simulink model "Clik_Jacobian_pseudoinverse"  (R2023b)
settings: Solver=VariableStepAuto  StartTime=0.0  StopTime=20  RelTol=1e-3
undefined symbols (not defined in the file): DiscIntNeverNeededParam, f_s
settings Model: Creator=Gianluca  LastModifiedBy=ANDREA
settings OptimizationCC: ReuseModelBlockBuffer=off
settings ModelReferenceCC: EnableRefExpFcnMdlSchedulingChecks=on

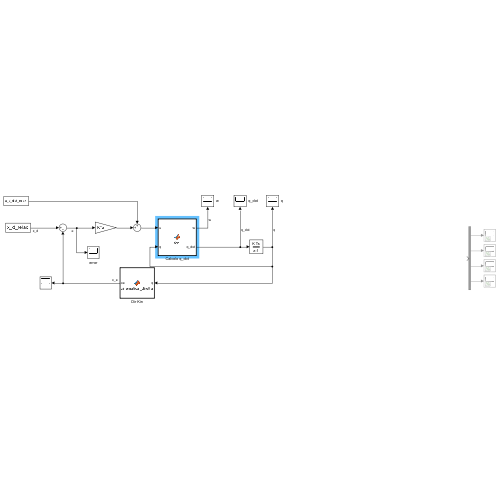
[thumbnail: Simulink's stored preview of the top-level diagram]
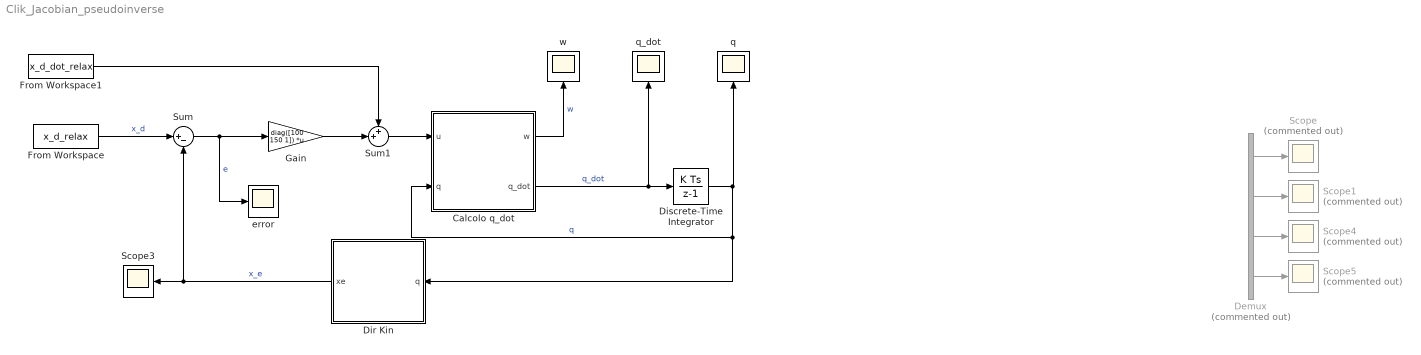
== system Clik_Jacobian_pseudoinverse ==
  "Calcolo q_dot " : MATLAB Function  TreatAsAtomicUnit=on
  Demux : Demux  Commented=on
  Dir Kin : MATLAB Function  TreatAsAtomicUnit=on
  Discrete-Time Integrator : DiscreteIntegrator  InitialCondition=[1.07216, -1.5708, 0.2, -0.49864 ]  SampleTime=1/f_s  ICPrevOutput=DiscIntNeverNeededParam  ICPrevScaledInput=DiscIntNeverNeededParam
  From Workspace : FromWorkspace  VariableName=x_d_relax  OutputAfterFinalValue=Holding final value
  From Workspace1 : FromWorkspace  VariableName=x_d_dot_relax
  Gain : Gain  Gain=diag([100 150 1])  Multiplication=Matrix(K*u)
  Scope{,1,4..5} (4 alike) : Scope  Commented=on
  Scope3 : Scope
  Sum : Sum  Inputs=|+-
  Sum1 : Sum  Inputs=++|
  error : Scope
  q : Scope
  q_dot : Scope
  w : Scope
  wires:
  Discrete-Time Integrator/1 -> q/1, Dir Kin/1(q), "Calcolo q_dot "/2(q)  "q"
  Gain/1 -> Sum1/2
  Sum1/1 -> "Calcolo q_dot "/1(u)
  "Calcolo q_dot "/2(q_dot) -> q_dot/1, Discrete-Time Integrator/1  "q_dot"
  Demux/1 -> Scope/1
  Demux/2 -> Scope1/1
  Demux/3 -> Scope4/1
  Sum/1 -> error/1, Gain/1  "e"
  "Calcolo q_dot "/1(w) -> w/1  "w"
  From Workspace/1 -> Sum/1  "x_d"
  Dir Kin/1(xe) -> Scope3/1, Sum/2  "x_e"
  Demux/4 -> Scope5/1
  From Workspace1/1 -> Sum1/1

== matlab function Clik_Jacobian_pseudoinverse/Calcolo q_dot  ==
  data: u input; q input; w output; q_dot output
function [w, q_dot] = fcn(u, q)
    
    J = [cos(q(1) + q(2))/2 + cos(q(1))/2       cos(q(1) + q(2))/2  0  0
         0                                      0                   -1 0
         1                                      1                   0  -1];

    q_0_dot = 100*[0, sqrt(2)*sin(2*q(2))/(8*sqrt(1-cos(2*q(2)))), 0, 0]';
    q_dot = pinv(J)*u+(eye(4)-pinv(J)*J)*q_0_dot;
    w = sqrt(det(J*J'));

end

== matlab function Clik_Jacobian_pseudoinverse/Dir Kin ==
  data: q input; xe output
function xe = cinematica_diretta(q)
    
    xe = [  0.5*sin(q(1))+0.5*sin(q(1)+q(2));
            1/2-q(3)
            q(1)+q(2)-q(4) ];

end
